simulink model "Signal_Processing"  (R2019b)
settings: Solver=FixedStepAuto  StartTime=0.0  StopTime=10  FixedStep=0.005  RelTol=1e-3
InitFcn:
  | load('BusDefinitions.mat')
settings Model: ExtModeTrigDuration=80  Creator=rjgoo  LastModifiedBy=rjgoo
settings DataIOCC: SaveFormat=StructureWithTime  ReturnWorkspaceOutputs=off
settings OptimizationCC: PassReuseOutputArgsThreshold=0  MaxStackSize=64
settings DebuggingCC: ParameterTunabilityLossMsg=error  ArithmeticOperatorsInVariantConditions=warning
settings HardwareCC: ProdBitPerPointer=32  ProdBitPerSizeT=32  ProdBitPerPtrDiffT=32  ProdLargestAtomicInteger=Long  ProdWordSize=32  ProdHWDeviceType=ARM Compatible->ARM 9
settings SFSimCC: SimUseLocalCustomCode=off  MATLABDynamicMemAlloc=off  CustomCodeUndefinedFunction=UseInterfaceOnly
settings RTWCC: SystemTargetFile=ert.tlc  HardwareBoard=PARROT Mambo  TLCOptions=-aInlineSetEventsForThisBaseRateFcn=TLC_FALSE -aSuppressMultiTaskScheduler=TLC_FALSE -aRateBasedStepFcn=1  TemplateMakefile=ert_default_tmf  GenerateReport=on  RTWUseLocalCustomCode=off  Toolchain=Sourcery G++ Lite GNU Toolchain for Drones  LaunchReport=on
settings CodeAppCC: ForceParamTrailComments=on  OperatorAnnotations=on  StateflowObjectComments=on
settings ERTTargetCC: ERTCustomFileBanners=off  MatFileLogging=on  SupportContinuousTime=on  SupportNonInlinedSFcns=on  RemoveResetFunc=off  ModelStepFunctionPrototypeControlCompliant=off

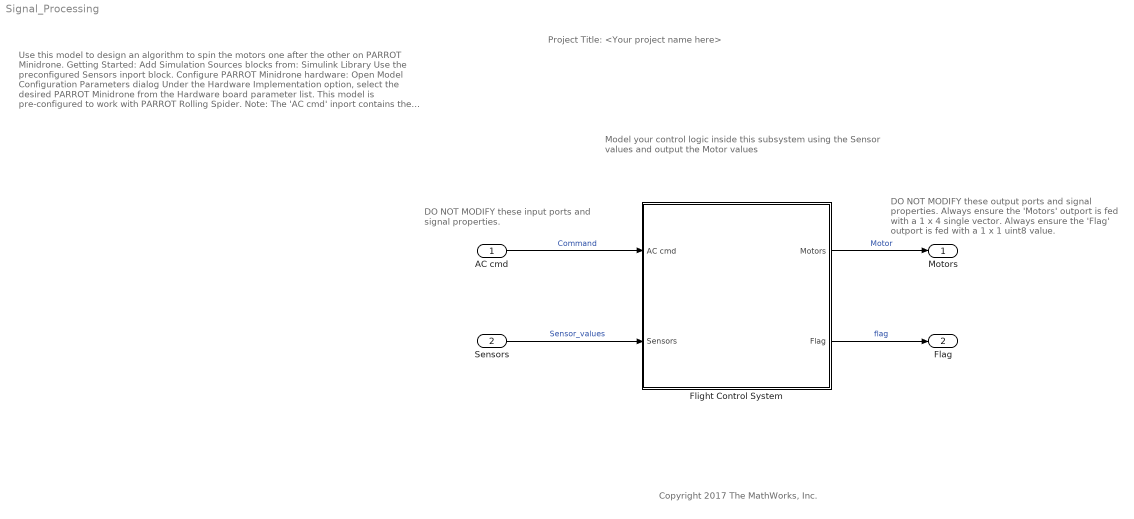
== system Signal_Processing ==
  note: Model your control logic inside this subsystem
      | using the Sensor values and output the
      | Motor values
  note: DO NOT MODIFY these output ports
      | and signal properties.
      |
      |
      |
      | Always ensure the 'Motors' outport
      | is fed with a 1 x 4 single vector.
      |
      |
      |
      |
      |
      | Always ensure the 'Flag' outport is
      | fed with a 1 x 1 uint8 value.
  note: DO NOT MODIFY these input
      | ports and signal properties.
  note: Copyright 2017 The MathWorks, Inc.
  note: Use this model to design an algorithm to spin the motors one
      | after the other on PARROT Minidrone.
      |
      | Getting Started:
      |
      | Add Simulation Sources blocks from:
      | Simulink Library
      | Use the preconfigured Sensors inport block.
      |
      | Configure PARROT Minidrone hardware:
      |
      | Open Model Configuration Parameters dialog
      |
      | Under the Hardware Implementation option, select the desired
      | PARROT Minidrone from the Hardware board parameter list.
      |
      | This model is pre-configured to work with PARROT Rolling Spider.
      |
      | Note:
      |
      | The 'AC cmd' inport contains the position and orientation
      | reference signals information.
      | The 'Sensors' inport contains data from accelerometer,
      | gyroscope, ultrasonic, pressure and optical flow data.
      | The 'Flag' outport can be used to model an error condition
      | which stops the drone.
      | The 'Motors' outport is fed with the speed values of the 4 motors.
      | Learn more:
      |
      | Simulink Subsystem
      | Simulink Buses
  note: Project Title: <Your project name here>
  AC cmd : Inport  OutDataTypeStr=Bus: CommandBus  BusOutputAsStruct=on
  Sensors : Inport  Port=2  OutDataTypeStr=Bus: SensorsBus  BusOutputAsStruct=on
  Flight Control System : Subsystem
  Motors : Outport  OutDataTypeStr=single  PortDimensions=[1 4]  VectorParamsAs1DForOutWhenUnconnected=off
  Flag : Outport  Port=2  OutDataTypeStr=uint8  PortDimensions=1  VectorParamsAs1DForOutWhenUnconnected=off
  wires:
  Flight Control System/1(Motors) -> Motors/1  "Motor"
  AC cmd/1 -> Flight Control System/1(AC cmd)  "Command"
  Sensors/1 -> Flight Control System/2(Sensors)  "Sensor_values"
  Flight Control System/2(Flag) -> Flag/1  "flag"

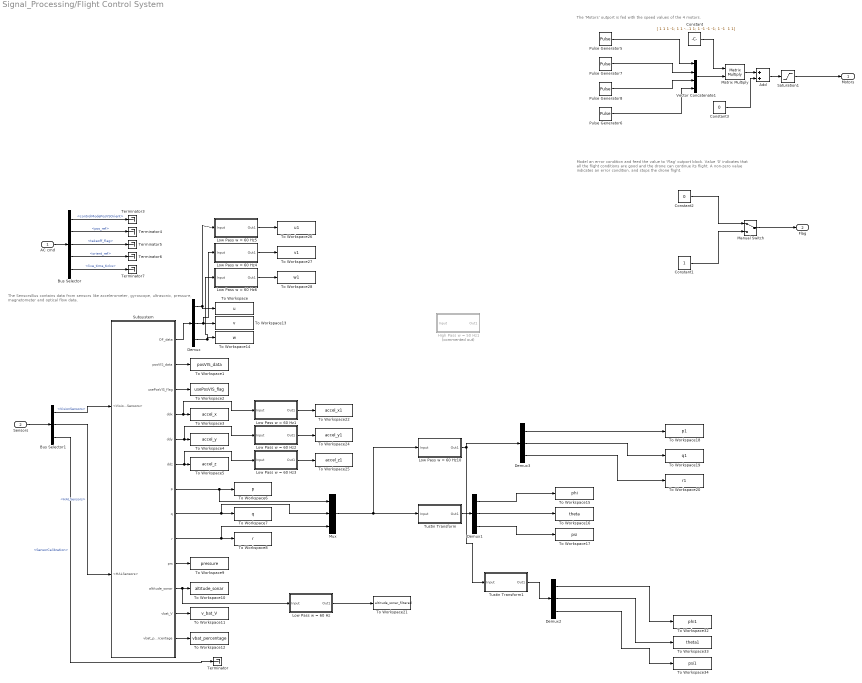
== system Signal_Processing/Flight Control System ==
  note: The 'Motors' outport is fed with the speed values of the 4 motors.
  note: Model an error condition and feed the value to 'Flag' outport block.
      | Value '0' indicates that all the flight conditions are good and the drone
      | can continue its flight.
      | A non-zero value indicates an error condition, and stops the drone
      | flight.
  note: The SensorsBus contains data from sensors like
      | accelerometer, gyroscope, ultrasonic, pressure,
      | magnetometer and optical flow data.
  AC cmd : Inport
  Sensors : Inport  Port=2
  Add : Sum
  Bus Selector : BusSelector  OutputSignals=controlModePosVSOrient,pos_ref,takeoff_flag,orient_ref,live_time_ticks
  Bus Selector1 : BusSelector  OutputSignals=VisionSensors,HALSensors,SensorCalibration
  Constant : Constant  Value="[ 1 1 1 -1; 1 1 -1 1; 1 -1 -1 -1; 1 -1  1 1]"
  Constant1 : Constant  OutDataTypeStr=uint8
  Constant2 : Constant  Value=0  OutDataTypeStr=uint8
  Constant3 : Constant  Value=0
  Demux{,1..3} (4 alike) : Demux  Outputs=3
  High Pass w = 50 Hz1 : Subsystem  Commented=on
  Low Pass w = 60 Hz : Subsystem
  Low Pass w = 60 Hz1 : Subsystem
  Low Pass w = 60 Hz10 : Subsystem
  Low Pass w = 60 Hz2 : Subsystem
  Low Pass w = 60 Hz3 : Subsystem
  Low Pass w = 60 Hz4 : Subsystem
  Low Pass w = 60 Hz5 : Subsystem
  Low Pass w = 60 Hz6 : Subsystem
  Manual Switch : ManualSwitch
  Matrix Multiply : Product  Multiplication=Matrix(*)
  Mux : Mux  Inputs=3
  Pulse Generator5 : DiscretePulseGenerator  PulseType=Time based  Amplitude=200  Period=20  PulseWidth=50  SampleTime=0.005
  Pulse Generator6 : DiscretePulseGenerator  PulseType=Time based  Amplitude=400  Period=16  PulseWidth=25  PhaseDelay=20  SampleTime=0.005
  Pulse Generator7 : DiscretePulseGenerator  PulseType=Time based  Amplitude=400  Period=16  PulseWidth=25  PhaseDelay=20  SampleTime=0.005
  Pulse Generator8 : DiscretePulseGenerator  PulseType=Time based  Amplitude=400  Period=16  PulseWidth=25  PhaseDelay=20  SampleTime=0.005
  Saturation1 : Saturate  UpperLimit=500  LowerLimit=0  OutDataTypeStr=single
  Subsystem : Subsystem
  Terminator{,3..7} (6 alike) : Terminator
  To Workspace : ToWorkspace  VariableName=u  SaveFormat=Structure With Time  SampleTime=0.005
  To Workspace1 : ToWorkspace  VariableName=posVIS_data  SaveFormat=Structure With Time  SampleTime=0.005
  To Workspace10 : ToWorkspace  VariableName=altitude_sonar  SaveFormat=Structure With Time  SampleTime=0.005
  To Workspace11 : ToWorkspace  VariableName=v_bat_V  SaveFormat=Structure With Time  SampleTime=0.005
  To Workspace12 : ToWorkspace  VariableName=vbat_percentage  SaveFormat=Structure With Time  SampleTime=0.005
  To Workspace13 : ToWorkspace  VariableName=v  SaveFormat=Structure With Time  SampleTime=0.005
  To Workspace14 : ToWorkspace  VariableName=w  SaveFormat=Structure With Time  SampleTime=0.005
  To Workspace15 : ToWorkspace  VariableName=phi  SaveFormat=Structure With Time  SampleTime=0.005
  To Workspace16 : ToWorkspace  VariableName=theta  SaveFormat=Structure With Time  SampleTime=0.005
  To Workspace17 : ToWorkspace  VariableName=psi  SaveFormat=Structure With Time  SampleTime=0.005
  To Workspace18 : ToWorkspace  VariableName=p1  SaveFormat=Structure With Time  SampleTime=0.005
  To Workspace19 : ToWorkspace  VariableName=q1  SaveFormat=Structure With Time  SampleTime=0.005
  To Workspace2 : ToWorkspace  VariableName=usePosVIS_flag  SaveFormat=Structure With Time  SampleTime=0.005
  To Workspace20 : ToWorkspace  VariableName=r1  SaveFormat=Structure With Time  SampleTime=0.005
  To Workspace21 : ToWorkspace  VariableName=altitude_sonar_filtered  SaveFormat=Structure With Time  SampleTime=0.005
  To Workspace22 : ToWorkspace  VariableName=accel_x1  SaveFormat=Structure With Time  SampleTime=0.005
  To Workspace24 : ToWorkspace  VariableName=accel_y1  SaveFormat=Structure With Time  SampleTime=0.005
  To Workspace25 : ToWorkspace  VariableName=accel_z1  SaveFormat=Structure With Time  SampleTime=0.005
  To Workspace26 : ToWorkspace  VariableName=u1  SaveFormat=Structure With Time  SampleTime=0.005
  To Workspace27 : ToWorkspace  VariableName=v1  SaveFormat=Structure With Time  SampleTime=0.005
  To Workspace28 : ToWorkspace  VariableName=w1  SaveFormat=Structure With Time  SampleTime=0.005
  To Workspace3 : ToWorkspace  VariableName=accel_x  SaveFormat=Structure With Time  SampleTime=0.005
  To Workspace32 : ToWorkspace  VariableName=phi1  SaveFormat=Structure With Time  SampleTime=0.005
  To Workspace33 : ToWorkspace  VariableName=theta1  SaveFormat=Structure With Time  SampleTime=0.005
  To Workspace34 : ToWorkspace  VariableName=psi1  SaveFormat=Structure With Time  SampleTime=0.005
  To Workspace4 : ToWorkspace  VariableName=accel_y  SaveFormat=Structure With Time  SampleTime=0.005
  To Workspace5 : ToWorkspace  VariableName=accel_z  SaveFormat=Structure With Time  SampleTime=0.005
  To Workspace6 : ToWorkspace  VariableName=p  SaveFormat=Structure With Time  SampleTime=0.005
  To Workspace7 : ToWorkspace  VariableName=q  SaveFormat=Structure With Time  SampleTime=0.005
  To Workspace8 : ToWorkspace  VariableName=r  SaveFormat=Structure With Time  SampleTime=0.005
  To Workspace9 : ToWorkspace  VariableName=pressure  SaveFormat=Structure With Time  SampleTime=0.005
  Tustin Transform : Subsystem
  Tustin Transform1 : Subsystem
  Vector Concatenate1 : Concatenate  NumInputs=4
  Motors : Outport  VectorParamsAs1DForOutWhenUnconnected=off
  Flag : Outport  Port=2  VectorParamsAs1DForOutWhenUnconnected=off
  wires:
  AC cmd/1 -> Bus Selector/1
  Sensors/1 -> Bus Selector1/1
  Bus Selector/1 -> Terminator3/1  "<controlModePosVSOrient>"
  Bus Selector/2 -> Terminator4/1  "<pos_ref>"
  Bus Selector/3 -> Terminator5/1  "<takeoff_flag>"
  Bus Selector/4 -> Terminator6/1  "<orient_ref>"
  Bus Selector/5 -> Terminator7/1  "<live_time_ticks>"
  Manual Switch/1 -> Flag/1
  Constant2/1 -> Manual Switch/1
  Constant1/1 -> Manual Switch/2
  Saturation1/1 -> Motors/1
  Bus Selector1/1 -> Subsystem/1(<VisionSensors>)  "<VisionSensors>"
  Bus Selector1/2 -> Subsystem/2(<HALSensors>)  "<HALSensors>"
  Subsystem/1(OF_data) -> Demux/1
  Subsystem/2(posVIS_data) -> To Workspace1/1
  Subsystem/3(usePosVIS_flag) -> To Workspace2/1
  Subsystem/4(ddx) -> Low Pass w = 60 Hz1/1(Input), To Workspace3/1
  Subsystem/5(ddy) -> Low Pass w = 60 Hz2/1(Input), To Workspace4/1
  Subsystem/6(ddz) -> Low Pass w = 60 Hz3/1(Input), To Workspace5/1
  Subsystem/7(p) -> Mux/1, To Workspace6/1
  Subsystem/9(r) -> Mux/3, To Workspace8/1
  Subsystem/10(prs) -> To Workspace9/1
  Subsystem/11(altitude_sonar) -> Low Pass w = 60 Hz/1(Input), To Workspace10/1
  Subsystem/12(vbat_V) -> To Workspace11/1
  Subsystem/13(vbat_percentage) -> To Workspace12/1
  Subsystem/8(q) -> Mux/2, To Workspace7/1
  Bus Selector1/3 -> Terminator/1  "<SensorCalibration>"
  Constant/1 -> Matrix Multiply/1
  Vector Concatenate1/1 -> Matrix Multiply/2
  Matrix Multiply/1 -> Add/1
  Add/1 -> Saturation1/1
  Constant3/1 -> Add/2
  Pulse Generator5/1 -> Vector Concatenate1/1
  Pulse Generator7/1 -> Vector Concatenate1/2
  Pulse Generator6/1 -> Vector Concatenate1/4
  Pulse Generator8/1 -> Vector Concatenate1/3
  Demux/2 -> Low Pass w = 60 Hz4/1(Input), To Workspace13/1
  Demux/3 -> Low Pass w = 60 Hz6/1(Input), To Workspace14/1
  Mux/1 -> Low Pass w = 60 Hz10/1(Input), Tustin Transform/1(Input)
  Tustin Transform/1(Out1) -> Demux1/1
  Demux1/1 -> To Workspace15/1
  Demux1/2 -> To Workspace16/1
  Demux1/3 -> To Workspace17/1
  Low Pass w = 60 Hz/1(Out1) -> To Workspace21/1
  Low Pass w = 60 Hz1/1(Out1) -> To Workspace22/1
  Low Pass w = 60 Hz2/1(Out1) -> To Workspace24/1
  Low Pass w = 60 Hz3/1(Out1) -> To Workspace25/1
  Low Pass w = 60 Hz6/1(Out1) -> To Workspace28/1
  Low Pass w = 60 Hz4/1(Out1) -> To Workspace27/1
  Low Pass w = 60 Hz5/1(Out1) -> To Workspace26/1
  Demux/1 -> Low Pass w = 60 Hz5/1(Input), To Workspace/1
  Demux2/1 -> To Workspace32/1
  Demux2/2 -> To Workspace33/1
  Demux2/3 -> To Workspace34/1
  Tustin Transform1/1(Out1) -> Demux2/1
  Demux3/1 -> To Workspace18/1
  Demux3/3 -> To Workspace20/1
  Demux3/2 -> To Workspace19/1
  Low Pass w = 60 Hz10/1(Out1) -> Tustin Transform1/1(Input), Demux3/1

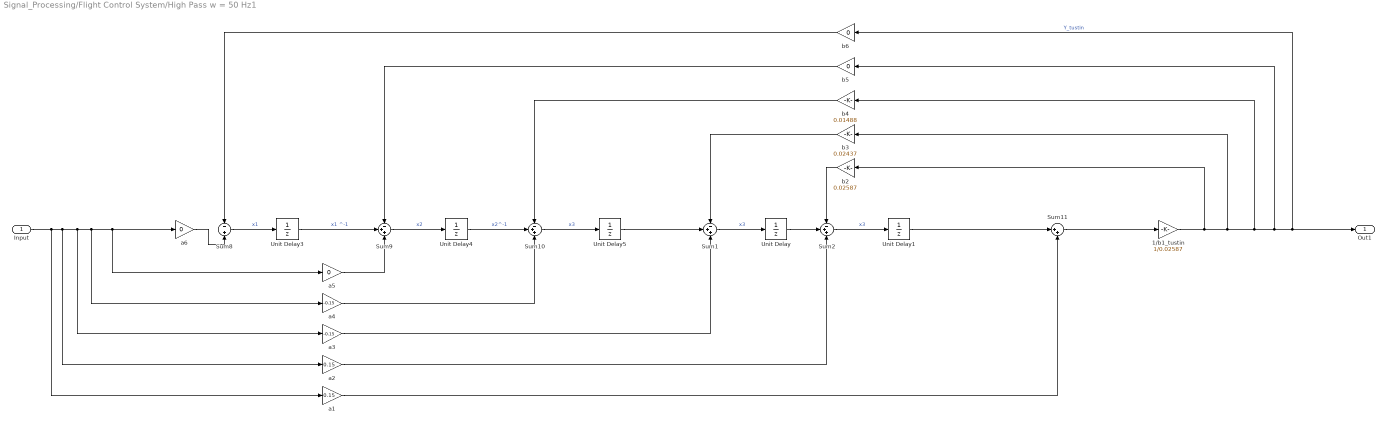
== system Signal_Processing/Flight Control System/High Pass w = 50 Hz1 ==
  Input : Inport
  1/b1_tustin : Gain  Gain=1/0.02587
  Sum{1..2,9..10} (4 alike) : Sum  Inputs=-++
  Sum11 : Sum  Inputs=|++
  Sum8 : Sum  Inputs=-|+
  Unit Delay : UnitDelay  SampleTime=-1  HasFrameUpgradeWarning=on
  Unit Delay1 : UnitDelay  SampleTime=-1  HasFrameUpgradeWarning=on
  Unit Delay3 : UnitDelay  SampleTime=.1  HasFrameUpgradeWarning=on
  Unit Delay4 : UnitDelay  SampleTime=0.1  HasFrameUpgradeWarning=on
  Unit Delay5 : UnitDelay  SampleTime=0.1  HasFrameUpgradeWarning=on
  a1 : Gain  Gain=0.15
  a2 : Gain  Gain=0.15
  a3 : Gain  Gain=-0.15
  "a4 " : Gain  Gain=-0.15
  a5 : Gain  Gain=0
  a6 : Gain  Gain=0
  b2 : Gain  Gain=0.02587
  b3 : Gain  Gain=0.02437
  b4 : Gain  Gain=0.01488
  b5 : Gain  Gain=0
  b6 : Gain  Gain=0
  Out1 : Outport
  wires:
  Sum8/1 -> Unit Delay3/1  "x1"
  Sum11/1 -> 1/b1_tustin/1
  Input/1 -> a1/1, a2/1, a3/1, "a4 "/1, a5/1, a6/1
  Sum9/1 -> Unit Delay4/1  "x2"
  Sum10/1 -> Unit Delay5/1  "x3"
  Unit Delay4/1 -> Sum10/2  "x2^-1"
  Unit Delay3/1 -> Sum9/2  "x1 ^-1"
  a6/1 -> Sum8/2
  1/b1_tustin/1 -> b2/1, b3/1, b4/1, b5/1, b6/1, Out1/1  "Y_tustin"
  Unit Delay5/1 -> Sum1/2
  Sum1/1 -> Unit Delay/1  "x3"
  Unit Delay/1 -> Sum2/2
  Sum2/1 -> Unit Delay1/1  "x3"
  Unit Delay1/1 -> Sum11/1
  b6/1 -> Sum8/1
  b5/1 -> Sum9/1
  b4/1 -> Sum10/1
  b3/1 -> Sum1/1
  b2/1 -> Sum2/1
  a1/1 -> Sum11/2
  a2/1 -> Sum2/3
  a3/1 -> Sum1/3
  "a4 "/1 -> Sum10/3
  a5/1 -> Sum9/3

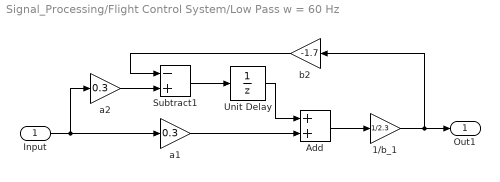
== system Signal_Processing/Flight Control System/Low Pass w = 60 Hz ==
  Input : Inport
  1/b_1 : Gain  Gain=1/2.3
  Add : Sum
  Subtract1 : Sum  Inputs=-+
  Unit Delay : UnitDelay  SampleTime=-1  HasFrameUpgradeWarning=on
  a1 : Gain  Gain=0.3
  a2 : Gain  Gain=0.3
  b2 : Gain  Gain=-1.7
  Out1 : Outport
  wires:
  Input/1 -> a1/1, a2/1
  1/b_1/1 -> Out1/1, b2/1
  b2/1 -> Subtract1/1
  a1/1 -> Add/2
  Subtract1/1 -> Unit Delay/1
  a2/1 -> Subtract1/2
  Unit Delay/1 -> Add/1
  Add/1 -> 1/b_1/1

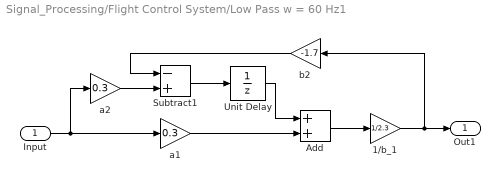
== system Signal_Processing/Flight Control System/Low Pass w = 60 Hz1 ==
  Input : Inport
  1/b_1 : Gain  Gain=1/2.3
  Add : Sum
  Subtract1 : Sum  Inputs=-+
  Unit Delay : UnitDelay  SampleTime=-1  HasFrameUpgradeWarning=on
  a1 : Gain  Gain=0.3
  a2 : Gain  Gain=0.3
  b2 : Gain  Gain=-1.7
  Out1 : Outport
  wires:
  Input/1 -> a1/1, a2/1
  1/b_1/1 -> Out1/1, b2/1
  b2/1 -> Subtract1/1
  a1/1 -> Add/2
  Subtract1/1 -> Unit Delay/1
  a2/1 -> Subtract1/2
  Unit Delay/1 -> Add/1
  Add/1 -> 1/b_1/1

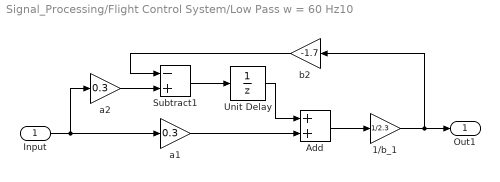
== system Signal_Processing/Flight Control System/Low Pass w = 60 Hz10 ==
  Input : Inport
  1/b_1 : Gain  Gain=1/2.3
  Add : Sum
  Subtract1 : Sum  Inputs=-+
  Unit Delay : UnitDelay  SampleTime=-1  HasFrameUpgradeWarning=on
  a1 : Gain  Gain=0.3
  a2 : Gain  Gain=0.3
  b2 : Gain  Gain=-1.7
  Out1 : Outport
  wires:
  Input/1 -> a1/1, a2/1
  1/b_1/1 -> Out1/1, b2/1
  b2/1 -> Subtract1/1
  a1/1 -> Add/2
  Subtract1/1 -> Unit Delay/1
  a2/1 -> Subtract1/2
  Unit Delay/1 -> Add/1
  Add/1 -> 1/b_1/1

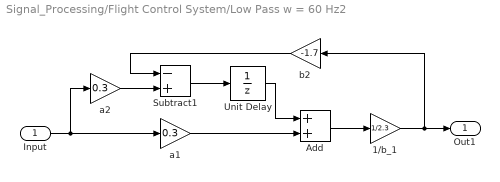
== system Signal_Processing/Flight Control System/Low Pass w = 60 Hz2 ==
  Input : Inport
  1/b_1 : Gain  Gain=1/2.3
  Add : Sum
  Subtract1 : Sum  Inputs=-+
  Unit Delay : UnitDelay  SampleTime=-1  HasFrameUpgradeWarning=on
  a1 : Gain  Gain=0.3
  a2 : Gain  Gain=0.3
  b2 : Gain  Gain=-1.7
  Out1 : Outport
  wires:
  Input/1 -> a1/1, a2/1
  1/b_1/1 -> Out1/1, b2/1
  b2/1 -> Subtract1/1
  a1/1 -> Add/2
  Subtract1/1 -> Unit Delay/1
  a2/1 -> Subtract1/2
  Unit Delay/1 -> Add/1
  Add/1 -> 1/b_1/1

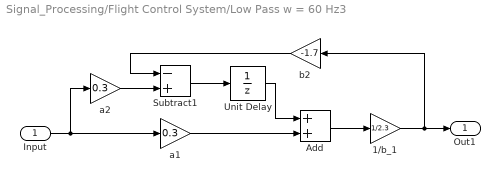
== system Signal_Processing/Flight Control System/Low Pass w = 60 Hz3 ==
  Input : Inport
  1/b_1 : Gain  Gain=1/2.3
  Add : Sum
  Subtract1 : Sum  Inputs=-+
  Unit Delay : UnitDelay  SampleTime=-1  HasFrameUpgradeWarning=on
  a1 : Gain  Gain=0.3
  a2 : Gain  Gain=0.3
  b2 : Gain  Gain=-1.7
  Out1 : Outport
  wires:
  Input/1 -> a1/1, a2/1
  1/b_1/1 -> Out1/1, b2/1
  b2/1 -> Subtract1/1
  a1/1 -> Add/2
  Subtract1/1 -> Unit Delay/1
  a2/1 -> Subtract1/2
  Unit Delay/1 -> Add/1
  Add/1 -> 1/b_1/1

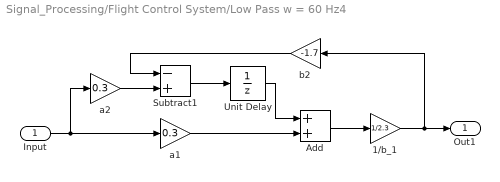
== system Signal_Processing/Flight Control System/Low Pass w = 60 Hz4 ==
  Input : Inport
  1/b_1 : Gain  Gain=1/2.3
  Add : Sum
  Subtract1 : Sum  Inputs=-+
  Unit Delay : UnitDelay  SampleTime=-1  HasFrameUpgradeWarning=on
  a1 : Gain  Gain=0.3
  a2 : Gain  Gain=0.3
  b2 : Gain  Gain=-1.7
  Out1 : Outport
  wires:
  Input/1 -> a1/1, a2/1
  1/b_1/1 -> Out1/1, b2/1
  b2/1 -> Subtract1/1
  a1/1 -> Add/2
  Subtract1/1 -> Unit Delay/1
  a2/1 -> Subtract1/2
  Unit Delay/1 -> Add/1
  Add/1 -> 1/b_1/1

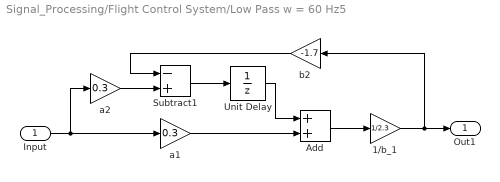
== system Signal_Processing/Flight Control System/Low Pass w = 60 Hz5 ==
  Input : Inport
  1/b_1 : Gain  Gain=1/2.3
  Add : Sum
  Subtract1 : Sum  Inputs=-+
  Unit Delay : UnitDelay  SampleTime=-1  HasFrameUpgradeWarning=on
  a1 : Gain  Gain=0.3
  a2 : Gain  Gain=0.3
  b2 : Gain  Gain=-1.7
  Out1 : Outport
  wires:
  Input/1 -> a1/1, a2/1
  1/b_1/1 -> Out1/1, b2/1
  b2/1 -> Subtract1/1
  a1/1 -> Add/2
  Subtract1/1 -> Unit Delay/1
  a2/1 -> Subtract1/2
  Unit Delay/1 -> Add/1
  Add/1 -> 1/b_1/1

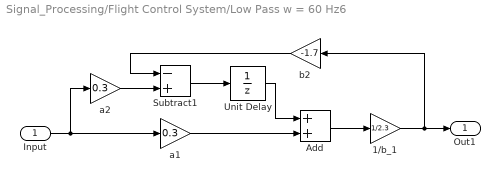
== system Signal_Processing/Flight Control System/Low Pass w = 60 Hz6 ==
  Input : Inport
  1/b_1 : Gain  Gain=1/2.3
  Add : Sum
  Subtract1 : Sum  Inputs=-+
  Unit Delay : UnitDelay  SampleTime=-1  HasFrameUpgradeWarning=on
  a1 : Gain  Gain=0.3
  a2 : Gain  Gain=0.3
  b2 : Gain  Gain=-1.7
  Out1 : Outport
  wires:
  Input/1 -> a1/1, a2/1
  1/b_1/1 -> Out1/1, b2/1
  b2/1 -> Subtract1/1
  a1/1 -> Add/2
  Subtract1/1 -> Unit Delay/1
  a2/1 -> Subtract1/2
  Unit Delay/1 -> Add/1
  Add/1 -> 1/b_1/1

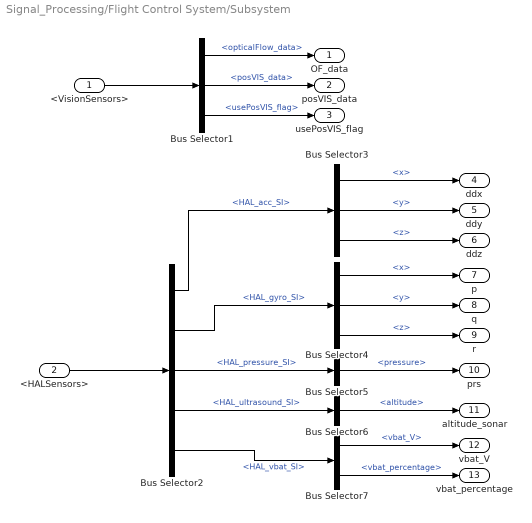
== system Signal_Processing/Flight Control System/Subsystem ==
  <VisionSensors> : Inport
  <HALSensors> : Inport  Port=2
  Bus Selector1 : BusSelector  OutputSignals=opticalFlow_data,posVIS_data,usePosVIS_flag
  Bus Selector2 : BusSelector  OutputSignals=HAL_acc_SI,HAL_gyro_SI,HAL_pressure_SI,HAL_ultrasound_SI,HAL_vbat_SI
  Bus Selector3 : BusSelector  OutputSignals=x,y,z
  Bus Selector4 : BusSelector  OutputSignals=x,y,z
  Bus Selector5 : BusSelector  OutputSignals=pressure
  Bus Selector6 : BusSelector  OutputSignals=altitude
  Bus Selector7 : BusSelector  OutputSignals=vbat_V,vbat_percentage
  OF_data : Outport  VectorParamsAs1DForOutWhenUnconnected=off
  posVIS_data : Outport  Port=2  VectorParamsAs1DForOutWhenUnconnected=off
  usePosVIS_flag : Outport  Port=3  VectorParamsAs1DForOutWhenUnconnected=off
  ddx : Outport  Port=4  VectorParamsAs1DForOutWhenUnconnected=off
  ddy : Outport  Port=5  VectorParamsAs1DForOutWhenUnconnected=off
  ddz : Outport  Port=6  VectorParamsAs1DForOutWhenUnconnected=off
  p : Outport  Port=7  VectorParamsAs1DForOutWhenUnconnected=off
  q : Outport  Port=8  VectorParamsAs1DForOutWhenUnconnected=off
  r : Outport  Port=9  VectorParamsAs1DForOutWhenUnconnected=off
  prs : Outport  Port=10  VectorParamsAs1DForOutWhenUnconnected=off
  altitude_sonar : Outport  Port=11  VectorParamsAs1DForOutWhenUnconnected=off
  vbat_V : Outport  Port=12  VectorParamsAs1DForOutWhenUnconnected=off
  vbat_percentage : Outport  Port=13  VectorParamsAs1DForOutWhenUnconnected=off
  wires:
  <VisionSensors>/1 -> Bus Selector1/1
  <HALSensors>/1 -> Bus Selector2/1
  Bus Selector1/1 -> OF_data/1  "<opticalFlow_data>"
  Bus Selector1/2 -> posVIS_data/1  "<posVIS_data>"
  Bus Selector1/3 -> usePosVIS_flag/1  "<usePosVIS_flag>"
  Bus Selector2/1 -> Bus Selector3/1  "<HAL_acc_SI>"
  Bus Selector2/2 -> Bus Selector4/1  "<HAL_gyro_SI>"
  Bus Selector2/3 -> Bus Selector5/1  "<HAL_pressure_SI>"
  Bus Selector2/4 -> Bus Selector6/1  "<HAL_ultrasound_SI>"
  Bus Selector2/5 -> Bus Selector7/1  "<HAL_vbat_SI>"
  Bus Selector3/1 -> ddx/1  "<x>"
  Bus Selector3/2 -> ddy/1  "<y>"
  Bus Selector3/3 -> ddz/1  "<z>"
  Bus Selector4/2 -> q/1  "<y>"
  Bus Selector4/1 -> p/1  "<x>"
  Bus Selector4/3 -> r/1  "<z>"
  Bus Selector5/1 -> prs/1  "<pressure>"
  Bus Selector6/1 -> altitude_sonar/1  "<altitude>"
  Bus Selector7/1 -> vbat_V/1  "<vbat_V>"
  Bus Selector7/2 -> vbat_percentage/1  "<vbat_percentage>"

== system Signal_Processing/Flight Control System/Tustin Transform ==
  Input : Inport
  1/b_1 : Gain  Gain=1/2
  Add : Sum
  Subtract : Sum  Inputs=-+
  Unit Delay : UnitDelay  SampleTime=-1  HasFrameUpgradeWarning=on
  a1 : Gain  Gain=0.005
  a2 : Gain  Gain=0.005
  b2 : Gain  Gain=-2
  Out1 : Outport
  wires:
  Unit Delay/1 -> Add/1
  Add/1 -> 1/b_1/1
  Subtract/1 -> Unit Delay/1
  1/b_1/1 -> Out1/1, b2/1
  a2/1 -> Subtract/2
  b2/1 -> Subtract/1
  Input/1 -> a1/1, a2/1
  a1/1 -> Add/2

== system Signal_Processing/Flight Control System/Tustin Transform1 ==
  Input : Inport
  1/b_1 : Gain  Gain=1/2
  Add : Sum
  Subtract : Sum  Inputs=-+
  Unit Delay : UnitDelay  SampleTime=-1  HasFrameUpgradeWarning=on
  a1 : Gain  Gain=0.005
  a2 : Gain  Gain=0.005
  b2 : Gain  Gain=-2
  Out1 : Outport
  wires:
  Unit Delay/1 -> Add/1
  Add/1 -> 1/b_1/1
  Subtract/1 -> Unit Delay/1
  1/b_1/1 -> Out1/1, b2/1
  a2/1 -> Subtract/2
  b2/1 -> Subtract/1
  Input/1 -> a1/1, a2/1
  a1/1 -> Add/2
